simulink model "test"  (Simulink 7.8)
settings: Solver=ode3  StartTime=0.0  StopTime=inf  FixedStep=0.01  RelTol=1e-3
settings Model: Creator=Voytik  LastModifiedBy=Voytik
settings OptimizationCC: OptimizeModelRefInitCode=on  LifeSpan=Inf
settings RTWCC: SystemTargetFile=ert.tlc  GenerateMakefile=off  TemplateMakefile=ert_default_tmf  Description=Embedded Coder  ProcessScript=ert_make_rtw_hook
settings CodeAppCC: IgnoreCustomStorageClasses=off
settings ERTTargetCC: MultiwordLength=2048  GenerateSampleERTMain=on  ERTCustomFileTemplate=example_file_process.tlc  ConvertIfToSwitch=off  SuppressUnreachableDefaultCases=off

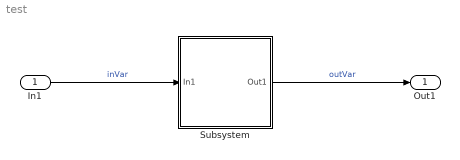
== system test ==
  In1 : Inport  OutDataTypeStr=double
  Subsystem : Subsystem
  Out1 : Outport  OutDataTypeStr=double
  wires:
  In1/1 -> Subsystem/1(In1)  "inVar"
  Subsystem/1(Out1) -> Out1/1  "outVar"

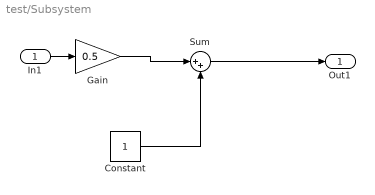
== system test/Subsystem ==
  In1 : Inport
  Constant : Constant
  Gain : Gain  Gain=0.5
  Sum : Sum  Inputs=|++
  Out1 : Outport
  wires:
  Gain/1 -> Sum/1
  Constant/1 -> Sum/2
  In1/1 -> Gain/1
  Sum/1 -> Out1/1
